simulink model "exampleStorage_hx_tube"  (R2016b)
settings: Solver=ode45  StartTime=0.0  StopTime=4*3600-0.1  RelTol=1e-3  EnableMultiTasking=on
libraries: carnot x15, simulink x4
settings Model: Creator=drhf  LastModifiedBy=drhf
settings DataIOCC: LimitDataPoints=on  SaveFormat=Array
settings OptimizationCC: ExpressionDepthLimit=2147483647  LifeSpan=inf
settings DebuggingCC: UnderspecifiedInitializationDetection=Classic  MergeDetectMultiDrivingBlocksExec=none  SolverPrmCheckMsg=warning  StateNameClashWarn=warning  SFUnexpectedBacktrackingDiag=warning  SFNoUnconditionalDefaultTransitionDiag=warning  SFExecutionAtInitializationDiag=none
settings HardwareCC: ProdBitPerPointer=32  ProdBitPerSizeT=32  ProdBitPerPtrDiffT=32  ProdLargestAtomicFloat=None  ProdIntDivRoundTo=Undefined  ProdEndianess=Unspecified  ProdWordSize=32  ProdHWDeviceType=32-bit Generic
settings ModelReferenceCC: PropagateSignalLabelsOutOfModel=off
settings GRTTargetCC: TargetLangStandard=C89/C90 (ANSI)  GeneratePreprocessorConditionals=Disable all  CombineOutputUpdateFcns=off  GRTInterface=on
settings ConfigComp: CovMetricSettings=dw  CovHtmlReporting=on  CovSaveCumulativeToWorkspaceVar=on  CovSaveSingleToWorkspaceVar=on  CovExternalEMLEnable=off

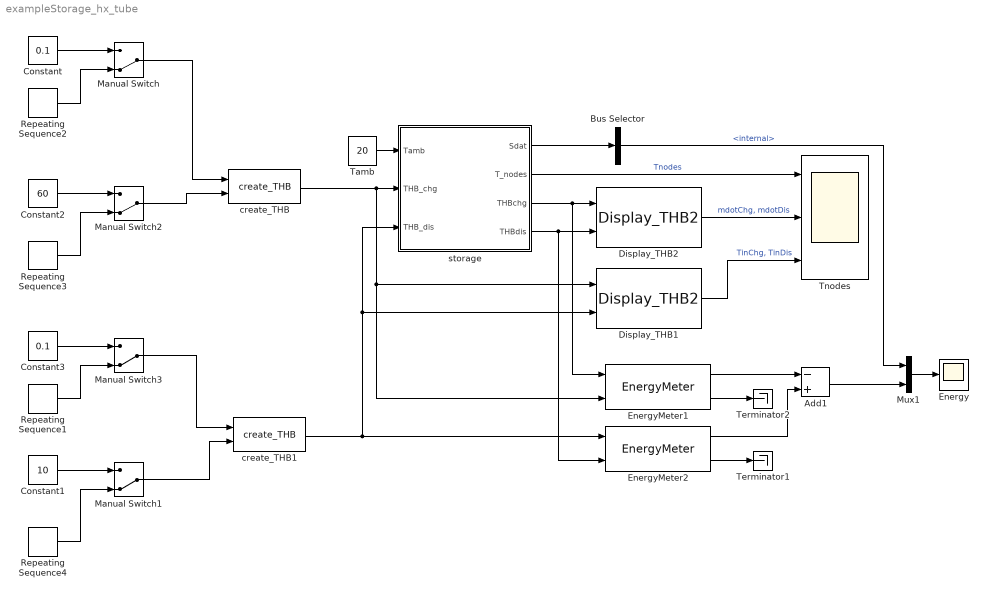
== system exampleStorage_hx_tube ==
  Add1 : Sum  Inputs=-+
  Bus Selector : BusSelector  OutputSignals=energy.internal
  Constant : Constant  Value=0.1
  Constant1 : Constant  Value=10
  Constant2 : Constant  Value=60
  Constant3 : Constant  Value=0.1
  Display_THB1 : carnot/Outputs/Display_THB2  t=on  m=off  p=off  id=off  mix=off  d=off
  Display_THB2 : carnot/Outputs/Display_THB2  t=off  m=on  p=off  id=off  mix=off  d=off
  Energy : Scope
  EnergyMeter1 : carnot/Control/EnergyMeter
  EnergyMeter2 : carnot/Control/EnergyMeter
  Manual Switch{,1..3} (4 alike) : ManualSwitch  CurrentSetting=0
  Mux1 : Mux  Inputs=2
  Repeating Sequence1 : simulink/Sources/Repeating Sequence  rep_seq_t=[0 1 1.1 2 2.1 3 3.1 4]*3600  rep_seq_y=[0 0 0 0 1 1 0 0]*0.05
  Repeating Sequence2 : simulink/Sources/Repeating Sequence  rep_seq_t=[0 1 1.1 2 2.1 3 3.1 4]*3600  rep_seq_y=[0 0 1 1 0 0 1 1]*0.1
  Repeating Sequence3 : simulink/Sources/Repeating Sequence  rep_seq_t=[0 1 1.1 2 2.1 3 3.1 4]*3600  rep_seq_y=[60 60 60 30 30 30 60 60]
  Repeating Sequence4 : simulink/Sources/Repeating Sequence  rep_seq_t=[0 1 1.1 2 2.1 3 3.1 4]*3600  rep_seq_y=[10 10 10 10 10 40 10 10]
  Tamb : Constant  Value=20
  Terminator1 : Terminator
  Terminator2 : Terminator
  Tnodes : Scope  NumInputPorts=3
  create_THB : carnot/Source/Simple/create_THB  p=1e5  fluid=Water  mix=0  mix2=0  mix3=0  dia=0  hgt=0  mID=No Pressure Drop
  create_THB1 : carnot/Source/Simple/create_THB  p=1e5  fluid=Water  mix=0  mix2=0  mix3=0  dia=0  hgt=0  mID=No Pressure Drop
  storage : Subsystem  mask(Multiport Storage){uloss=0, ubot=0, utop=0, cond=1, tini=[15:5:60], volume=0.3, dia=0.5, pos=standing cylinder, nconnect=2, nodes=10, mpoints=10}
      mask prompts: uloss "Heat loss coefficient cylinder wall in W/(m²K)"; ubot "Heat loss coefficient bottom in W/(m²K)"; utop "Heat loss coefficient top cover in W/(m²K)"; cond "Effective vertical conductivity in W/(m*K)"; tini "Initial temperature (vector or scalar) in °C"; volume "Volume in m³"; dia "Diameter in m"; pos "Position"; nconnect "Number of connections"; nodes "Number of nodes"; mpoints "Number of measurement points"
      mask help:
      | The volmue of the cylindrical storage is divided in a number "nodes" of horizontal slices (1xN-node model). For each node the energy balance equation is solved.
      | Look under mask to set the ports types and properties.
      mask init:
      | standing = pos-1;
      | 
      | if standing
      |     dh = volume/(0.25*dia^2*pi*nodes);
      | else
      |     dh = dia/nodes;
      | end
      | 
      | % height = 0.5*dh : dh : dh*nodes;
      | height = dh*nodes;
      | 
      | mpoints = max(mpoints,1);
      | mpts = round(nodes/mpoints/2:nodes/mpoints:nodes);
      mask Help: eval('man(''storage_multiport'')')
      mask TypeOptions pos: lying cylinder | standing cylinder
      mask Display: plot(10,10,90,100,[40,40,45,55,60,60,55,45,40],[84,36,30,30,36,84,90,90,84],[40,35],[77,77],[64,60],[77,77],[40,35],[42,42],[64,60],[42,42])
  wires:
  Bus Selector/1 -> Mux1/1  "<internal>"
  Tamb/1 -> storage/1(Tamb)
  create_THB/1 -> Display_THB1/1, EnergyMeter1/2, storage/2(THB_chg)
  create_THB1/1 -> storage/3(THB_dis), Display_THB1/2, EnergyMeter2/1
  storage/1(Sdat) -> Bus Selector/1
  storage/2(T_nodes) -> Tnodes/1  "Tnodes"
  storage/3(THBchg) -> Display_THB2/1, EnergyMeter1/1
  storage/4(THBdis) -> Display_THB2/2, EnergyMeter2/2
  Display_THB2/1 -> Tnodes/2  "mdotChg, mdotDis"
  Mux1/1 -> Energy/1
  EnergyMeter2/2 -> Terminator1/1
  Manual Switch3/1 -> create_THB1/1
  Manual Switch1/1 -> create_THB1/2
  Manual Switch/1 -> create_THB/1
  Constant/1 -> Manual Switch/1
  Constant1/1 -> Manual Switch1/1
  EnergyMeter1/2 -> Terminator2/1
  Add1/1 -> Mux1/2
  EnergyMeter2/1 -> Add1/2
  EnergyMeter1/1 -> Add1/1
  Constant2/1 -> Manual Switch2/1
  Repeating Sequence3/1 -> Manual Switch2/2
  Manual Switch2/1 -> create_THB/2
  Display_THB1/1 -> Tnodes/3  "TinChg, TinDis"
  Constant3/1 -> Manual Switch3/1
  Repeating Sequence4/1 -> Manual Switch1/2
  Repeating Sequence2/1 -> Manual Switch/2
  Repeating Sequence1/1 -> Manual Switch3/2

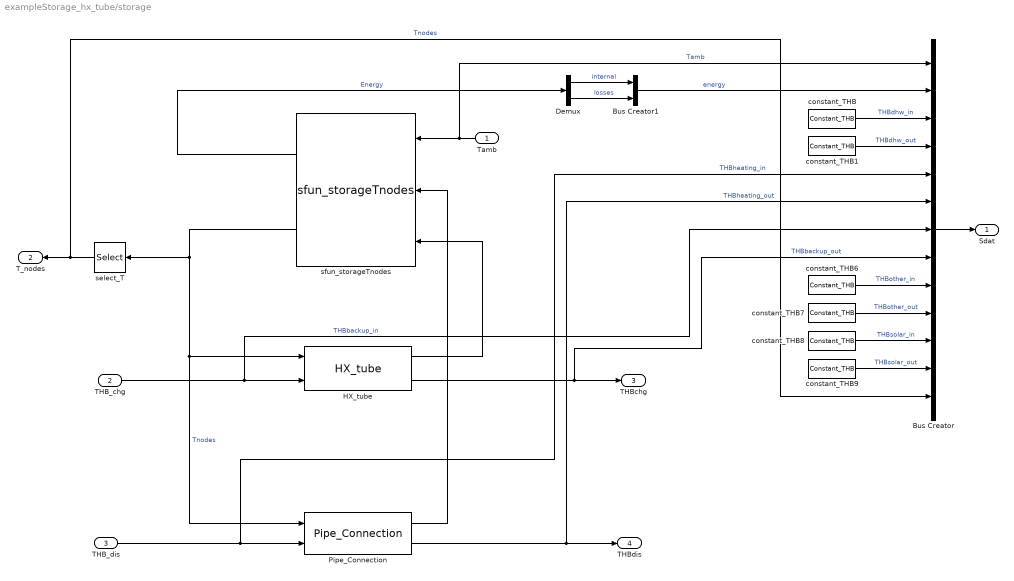
== system exampleStorage_hx_tube/storage ==
  Tamb : Inport
  THB_chg : Inport  Port=2
  THB_dis : Inport  Port=3
  Bus Creator : BusCreator  Inputs=13
  Bus Creator1 : BusCreator  Inputs=2
  Demux : Demux  Outputs=2
  HX_tube : carnot/Storage/Thermal/Storage_Ports/HX_tube  h_in=0.5  h_out=0  hgt=1.5  dpipe=0.03  swall=0.001  lpipe=10  cond=50  height=-0.75  dplin=100  dpqua=100  nodes=10
  Pipe_Connection : carnot/Storage/Thermal/Storage_Ports/Pipe_Connection  h_in=0  h_out=1  hgt=1  dia=0.03  height=1  nodes=nodes
  constant_THB{,1,6..9} (6 alike) : carnot/Source/Simple/Constant_THB  t=20  mdot=0  p=1e5  mID=No Pressure Drop  fluid=Water  mix=0  mix2=0  mix3=0  dia=0.02  hgt=0
  select_T : Selector  InputPortWidth=nodes  IndexOptions=Index vector (dialog)  Indices=mpts  OutputSizes=1
  sfun_storageTnodes : carnot/Basic/Thermal_Models/sfun_storageTnodes  uloss=uloss  ubot=ubot  utop=utop  cond=cond  volume=volume  dia=dia  standing=standing cylinder  tini=tini  nodes=nodes  nconnect=2  elimthermocline=2  condinvtc=1e5
  Sdat : Outport
  T_nodes : Outport  Port=2
  THBchg : Outport  Port=3
  THBdis : Outport  Port=4
  wires:
  Bus Creator1/1 -> Bus Creator/2  "energy"
  Demux/2 -> Bus Creator1/2  "losses"
  Demux/1 -> Bus Creator1/1  "internal"
  HX_tube/1 -> sfun_storageTnodes/3
  HX_tube/2 -> Bus Creator/8, THBchg/1  "THBbackup_out"
  THB_chg/1 -> HX_tube/2, Bus Creator/7  "THBbackup_in"
  constant_THB6/1 -> Bus Creator/9  "THBother_in"
  constant_THB7/1 -> Bus Creator/10  "THBother_out"
  constant_THB8/1 -> Bus Creator/11  "THBsolar_in"
  constant_THB9/1 -> Bus Creator/12  "THBsolar_out"
  Bus Creator/1 -> Sdat/1
  constant_THB/1 -> Bus Creator/3  "THBdhw_in"
  constant_THB1/1 -> Bus Creator/4  "THBdhw_out"
  sfun_storageTnodes/2 -> HX_tube/1, Pipe_Connection/1, select_T/1  "Tnodes"
  sfun_storageTnodes/1 -> Demux/1  "Energy"
  select_T/1 -> Bus Creator/13, T_nodes/1  "Tnodes"
  Pipe_Connection/1 -> sfun_storageTnodes/2
  Pipe_Connection/2 -> Bus Creator/6, THBdis/1  "THBheating_out"
  THB_dis/1 -> Pipe_Connection/2, Bus Creator/5  "THBheating_in"
  Tamb/1 -> Bus Creator/1, sfun_storageTnodes/1  "Tamb"
